simulink model "fig7_61"  (Simulink 6.1)
settings: Solver=ode45  SolverMode=SingleTasking  StartTime=0.0  StopTime=30  RelTol=1e-3  AbsTol=1e-6
CloseFcn:
  | ;slview('closediagram',bdroot);;slview('closediagram',bdroot);
settings Model: LastModifiedBy=abbas  ExtModeTrigMode=oneshot  ExtModeArmWhenConnect=off  ExtModeAutoUpdateStatusClock=off
settings DataIOCC: LimitDataPoints=off
settings OptimizationCC: BlockReduction=off  BooleanDataType=off
settings HardwareCC: TargetUnknown=on
settings STFCustomTargetCC: TargetFcnLib=ansi_tfl_tmw.mat  GenFloatMathFcnCalls=ANSI_C  ModelReferenceCompliant=off  SystemTargetFile=grt.tlc

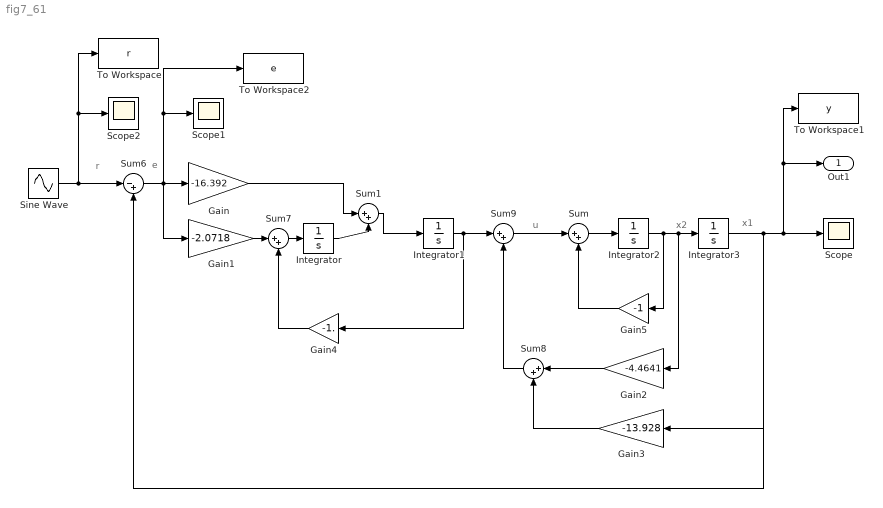
== system fig7_61 ==
  note: e
  note: u
  note: x2
  note: x1
  note: r
  Gain : Gain  Gain=-16.392  SaturateOnIntegerOverflow=on
  Gain1 : Gain  Gain=-2.0718  SaturateOnIntegerOverflow=on
  Gain2 : Gain  Orientation=left  Gain=-4.4641  SaturateOnIntegerOverflow=on
  Gain3 : Gain  Orientation=left  Gain=-13.928  SaturateOnIntegerOverflow=on
  Gain4 : Gain  Orientation=left  Gain=-1.  SaturateOnIntegerOverflow=on
  Gain5 : Gain  Orientation=left  Gain=-1  SaturateOnIntegerOverflow=on
  Integrator{,1..3} (4 alike) : Integrator
  Scope : Scope
      settings: TickLabels=on  DataFormat=Array
  Scope1 : Scope
      settings: TickLabels=on  DataFormat=Array
  Scope2 : Scope
  Sine Wave : Sin  SampleTime=.01
  Sum{,1,7,9} (4 alike) : Sum  Inputs=|++  SaturateOnIntegerOverflow=on  InputSameDT=on
  Sum6 : Sum  Inputs=|-+  SaturateOnIntegerOverflow=on  InputSameDT=on
  Sum8 : Sum  Orientation=left  Inputs=|++  SaturateOnIntegerOverflow=on  InputSameDT=on
  To Workspace : ToWorkspace  VariableName=r  SampleTime=.01  SaveFormat=Array
  To Workspace1 : ToWorkspace  VariableName=y  SampleTime=0.01  SaveFormat=Array
  To Workspace2 : ToWorkspace  VariableName=e  SampleTime=0.01  SaveFormat=Array
  Out1 : Outport
  wires:
  Sum7/1 -> Integrator/1
  Gain/1 -> Sum1/1
  Sum1/1 -> Integrator1/1
  Sum/1 -> Integrator2/1
  Integrator2/1 -> Integrator3/1, Gain2/1, Gain5/1
  Sum6/1 -> Gain/1, Gain1/1, Scope1/1, To Workspace2/1
  Integrator3/1 -> Sum6/2, Scope/1, Out1/1, To Workspace1/1, Gain3/1
  Gain3/1 -> Sum8/2
  Gain2/1 -> Sum8/1
  Gain1/1 -> Sum7/1
  Sum8/1 -> Sum9/2
  Integrator/1 -> Sum1/2
  Gain4/1 -> Sum7/2
  Gain5/1 -> Sum/2
  Integrator1/1 -> Gain4/1, Sum9/1
  Sine Wave/1 -> Sum6/1, Scope2/1, To Workspace/1
  Sum9/1 -> Sum/1
